simulink model "dynamic_range_compression"  (R2020b)
settings: Solver=FixedStepAuto  StartTime=0.0  StopTime=stop_time  RelTol=1e-3
values from neighbouring files (symbols this model uses):
  delay_memory_size = 2^system_delay_memory    [dynamic_range_compression_sim_init.m]    (also in test_FFT_to_gain_init.m)
  system_delay = gain_delay + accum_delay    [dynamic_range_compression_sim_init.m]    (also in test_FFT_to_gain_init.m)
libraries: hdlsllib x6
settings Model: Creator=t96f346  LastModifiedBy=conno
settings DataIOCC: SaveOutput=off  SaveTime=off  ReturnWorkspaceOutputs=off
settings ModelReferenceCC: ModelReferenceNumInstancesAllowed=Single

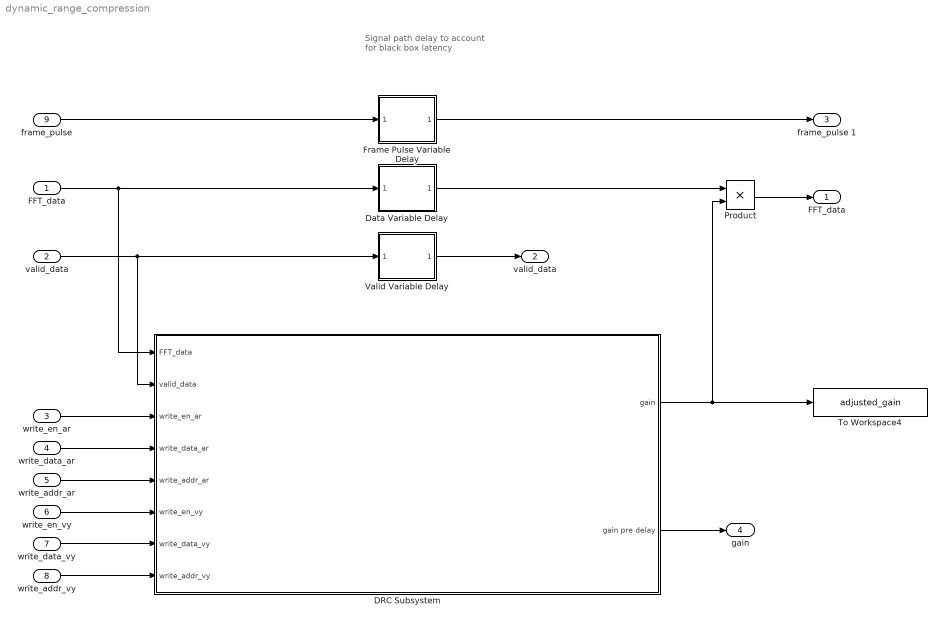
== system dynamic_range_compression ==
  note: Signal path delay to account for black box latency
  FFT_data : Inport  OutDataTypeStr=fixdt(1,40,32)  PortDimensions=[1 1]
      settings: SignalType=complex
  valid_data : Inport  Port=2  OutDataTypeStr=boolean  PortDimensions=[1 1]
  write_en_ar : Inport  Port=3  OutDataTypeStr=boolean  PortDimensions=[1 1]
  write_data_ar : Inport  Port=4  PortDimensions=[1 1]
  write_addr_ar : Inport  Port=5  OutDataTypeStr=uint8  PortDimensions=[1 1]
  write_en_vy : Inport  Port=6  OutDataTypeStr=boolean  PortDimensions=[1 1]
  write_data_vy : Inport  Port=7  OutDataTypeStr=fixdt(1,16,8)  PortDimensions=[1 1]
  write_addr_vy : Inport  Port=8  OutDataTypeStr=uint8  PortDimensions=[1 1]
  frame_pulse : Inport  Port=9  OutDataTypeStr=boolean  PortDimensions=[1 1]
  DRC Subsystem : Subsystem
  Data Variable Delay : Subsystem
  Frame Pulse Variable Delay : Subsystem
  Product : Product  OutDataTypeStr=fixdt(1,Wbits,Fbits)
  To Workspace4 : ToWorkspace  VariableName=adjusted_gain  SampleTime=-1
      settings: Save2DSignal=2-D array (concatenate along first dimension)
  Valid Variable Delay : Subsystem
  "FFT_data " : Outport  OutDataTypeStr=fixdt(1,40,32)  PortDimensions=1
      settings: SignalType=complex
  "valid_data " : Outport  Port=2  OutDataTypeStr=boolean  PortDimensions=1
  frame_pulse 1 : Outport  Port=3  OutDataTypeStr=boolean  PortDimensions=1
  gain : Outport  Port=4  PortDimensions=1
  wires:
  valid_data/1 -> Valid Variable Delay/1(data_in), DRC Subsystem/2(valid_data)
  FFT_data/1 -> Data Variable Delay/1(data_in), DRC Subsystem/1(FFT_data)
  Valid Variable Delay/1(rd_dout) -> "valid_data "/1
  write_en_ar/1 -> DRC Subsystem/3(write_en_ar)
  write_data_ar/1 -> DRC Subsystem/4(write_data_ar)
  write_addr_ar/1 -> DRC Subsystem/5(write_addr_ar)
  write_en_vy/1 -> DRC Subsystem/6(write_en_vy)
  write_data_vy/1 -> DRC Subsystem/7(write_data_vy)
  write_addr_vy/1 -> DRC Subsystem/8(write_addr_vy)
  DRC Subsystem/1("gain ") -> To Workspace4/1, Product/2
  Data Variable Delay/1(rd_dout) -> Product/1
  Product/1 -> "FFT_data "/1
  Frame Pulse Variable Delay/1(rd_dout) -> frame_pulse 1/1
  frame_pulse/1 -> Frame Pulse Variable Delay/1(data_in)
  DRC Subsystem/2(gain pre delay) -> gain/1

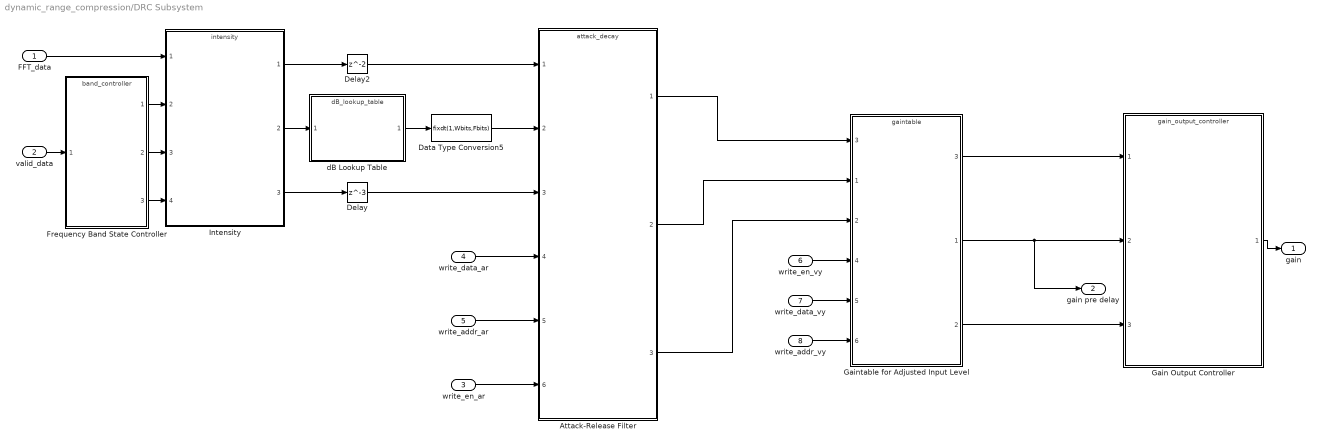
== system dynamic_range_compression/DRC Subsystem ==
  FFT_data : Inport
  valid_data : Inport  Port=2
  write_en_ar : Inport  Port=3
  write_data_ar : Inport  Port=4
  write_addr_ar : Inport  Port=5
  write_en_vy : Inport  Port=6
  write_data_vy : Inport  Port=7
  write_addr_vy : Inport  Port=8
  Attack-Release Filter : ModelReference  ModelNameDialog=attack_decay  SimulationMode=Normal  ModelReferenceVersion=2.75
  Data Type Conversion5 : DataTypeConversion  OutDataTypeStr=fixdt(1,Wbits,Fbits)
  Delay : Delay  DelayLength=3  InitialCondition=1
  Delay2 : Delay  InitialCondition=0
  Frequency Band State Controller : ModelReference  ModelNameDialog=band_controller.slx  SimulationMode=Normal  ModelReferenceVersion=2.34
  Gain Output Controller : ModelReference  ModelNameDialog=gain_output_controller.slx  SimulationMode=Normal  ModelReferenceVersion=2.28
  Gaintable for Adjusted Input Level : ModelReference  ModelNameDialog=gaintable  SimulationMode=Normal  ModelReferenceVersion=2.53
      settings: PortSchema="{\"entries\":[{\"content\":{\"sides\":[{\"content\":{\"connectorIds\":[\"In3\",\"In1\",\"In2\",\"In4\",\"In5\",\"In6\"]},\"type\":\"ConnectorPlacement.EquallySpacedRectSide\",\"uuid\":\"15a14a82-9bd7-4164-b619-b9bea276d1a9\"},{\"content\":{\"connectorIds\":[\"Out3\",\"Out1\",\"Out2\"],\"side\":\"RIGHT\"},\"type\":\"ConnectorPlacement.EquallySpacedRectSide\",\"uuid\":\"b762d0e2-66c7-466f-9495-f7c5ef747c3e\"},{\"content\":{\"connectorIds\":[],\"side\":\"TOP\"},\"type\":\"ConnectorPlacement.EquallySpacedRectSide\",\"uuid\":\"56b3a3d4-71ab-44aa-9541-48bc28b345d5\"},{\"content\":{\"connectorIds\":[],\"side\":\"HIDDEN\"},\"type\":\"ConnectorPlacement.EquallySpacedRectSide\",\"uuid\":\"17251429-5e91-446f-9fb8-583eb817a6ae\"}]},\"type\":\"ConnectorPlacement.EquallySpacedConnector\",\"uuid\":\"09e275fb-6840-46b7-a1cf-a56a9cd0acfa\"}],\"packageUris\":[\"http://schema.mathworks.com/mf0/Connector/R2020b\"],\"version\":\"1.0\"}"
  Intensity : ModelReference  ModelNameDialog=intensity  SimulationMode=Normal  ModelReferenceVersion=2.36
  dB Lookup Table : ModelReference  ModelNameDialog=dB_lookup_table  SimulationMode=Normal  ModelReferenceVersion=2.31
  "gain " : Outport
  gain pre delay : Outport  Port=2
  wires:
  Frequency Band State Controller/3 -> Intensity/4
  Gain Output Controller/1 -> "gain "/1
  valid_data/1 -> Frequency Band State Controller/1
  Intensity/2 -> dB Lookup Table/1
  FFT_data/1 -> Intensity/1
  Data Type Conversion5/1 -> Attack-Release Filter/2
  Gaintable for Adjusted Input Level/2 -> Gain Output Controller/3
  Frequency Band State Controller/1 -> Intensity/2
  Attack-Release Filter/2 -> Gaintable for Adjusted Input Level/1
  Delay/1 -> Attack-Release Filter/3
  Intensity/3 -> Delay/1
  Frequency Band State Controller/2 -> Intensity/3
  Delay2/1 -> Attack-Release Filter/1
  Intensity/1 -> Delay2/1
  Gaintable for Adjusted Input Level/1 -> Gain Output Controller/2, gain pre delay/1
  dB Lookup Table/1 -> Data Type Conversion5/1
  write_en_ar/1 -> Attack-Release Filter/6
  write_data_ar/1 -> Attack-Release Filter/4
  write_addr_ar/1 -> Attack-Release Filter/5
  Attack-Release Filter/3 -> Gaintable for Adjusted Input Level/2
  Attack-Release Filter/1 -> Gaintable for Adjusted Input Level/3
  Gaintable for Adjusted Input Level/3 -> Gain Output Controller/1
  write_en_vy/1 -> Gaintable for Adjusted Input Level/4
  write_data_vy/1 -> Gaintable for Adjusted Input Level/5
  write_addr_vy/1 -> Gaintable for Adjusted Input Level/6

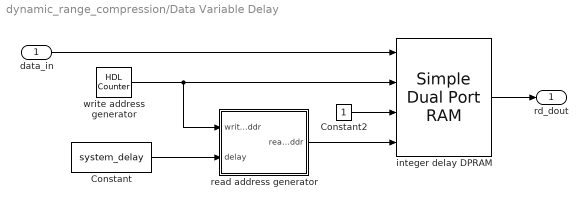
== system dynamic_range_compression/Data Variable Delay ==
  data_in : Inport
  Constant : Constant  Value=system_delay  OutDataTypeStr=uint8  SampleTime=-1
  Constant2 : Constant  OutDataTypeStr=Inherit: Inherit via back propagation  SampleTime=-1
  integer delay DPRAM : hdlsllib/HDL RAMs/Simple Dual Port RAM  ram_size=system_delay_memory
      settings: SourceProductBaseCode=SL
  read address generator : Subsystem
  write address generator : hdlsllib/Sources/HDL Counter  CountType=Count limited  CountInit=0  CountStep=1  CountMax=delay_memory_size - 1  CountFromType=Initial value  CountFrom=0  CountResetPort=off  CountLoadPort=off  CountEnbPort=off  CountDirPort=off  CountDataType=Unsigned  CountWordLen=system_delay_memory  CountFracLen=0  CountSampTime=-1
  rd_dout : Outport
  wires:
  read address generator/1(read_addr) -> integer delay DPRAM/4
  data_in/1 -> integer delay DPRAM/1
  Constant/1 -> read address generator/2(delay)
  integer delay DPRAM/1 -> rd_dout/1
  write address generator/1 -> read address generator/1(write_addr), integer delay DPRAM/2
  Constant2/1 -> integer delay DPRAM/3

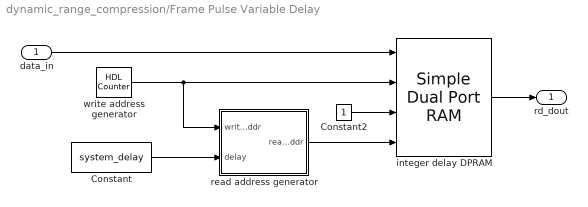
== system dynamic_range_compression/Frame Pulse Variable Delay ==
  data_in : Inport
  Constant : Constant  Value=system_delay  OutDataTypeStr=uint8  SampleTime=-1
  Constant2 : Constant  OutDataTypeStr=Inherit: Inherit via back propagation  SampleTime=-1
  integer delay DPRAM : hdlsllib/HDL RAMs/Simple Dual Port RAM  ram_size=system_delay_memory
      settings: SourceProductBaseCode=SL
  read address generator : Subsystem
  write address generator : hdlsllib/Sources/HDL Counter  CountType=Count limited  CountInit=0  CountStep=1  CountMax=delay_memory_size - 1  CountFromType=Initial value  CountFrom=0  CountResetPort=off  CountLoadPort=off  CountEnbPort=off  CountDirPort=off  CountDataType=Unsigned  CountWordLen=system_delay_memory  CountFracLen=0  CountSampTime=-1
  rd_dout : Outport
  wires:
  read address generator/1(read_addr) -> integer delay DPRAM/4
  data_in/1 -> integer delay DPRAM/1
  Constant/1 -> read address generator/2(delay)
  integer delay DPRAM/1 -> rd_dout/1
  write address generator/1 -> read address generator/1(write_addr), integer delay DPRAM/2
  Constant2/1 -> integer delay DPRAM/3

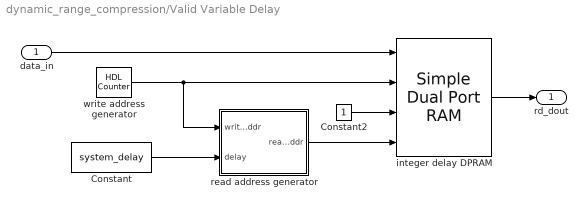
== system dynamic_range_compression/Valid Variable Delay ==
  data_in : Inport
  Constant : Constant  Value=system_delay  OutDataTypeStr=uint8  SampleTime=-1
  Constant2 : Constant  OutDataTypeStr=Inherit: Inherit via back propagation  SampleTime=-1
  integer delay DPRAM : hdlsllib/HDL RAMs/Simple Dual Port RAM  ram_size=system_delay_memory
      settings: SourceProductBaseCode=SL
  read address generator : Subsystem
  write address generator : hdlsllib/Sources/HDL Counter  CountType=Count limited  CountInit=0  CountStep=1  CountMax=delay_memory_size - 1  CountFromType=Initial value  CountFrom=0  CountResetPort=off  CountLoadPort=off  CountEnbPort=off  CountDirPort=off  CountDataType=Unsigned  CountWordLen=system_delay_memory  CountFracLen=0  CountSampTime=-1
  rd_dout : Outport
  wires:
  read address generator/1(read_addr) -> integer delay DPRAM/4
  data_in/1 -> integer delay DPRAM/1
  Constant/1 -> read address generator/2(delay)
  integer delay DPRAM/1 -> rd_dout/1
  write address generator/1 -> read address generator/1(write_addr), integer delay DPRAM/2
  Constant2/1 -> integer delay DPRAM/3

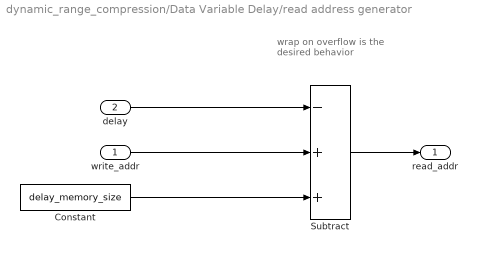
== system dynamic_range_compression/Data Variable Delay/read address generator ==
  note: wrap on overflow is the desired behavior
  write_addr : Inport
  delay : Inport  Port=2
  Constant : Constant  Value=delay_memory_size  SampleTime=-1
  Subtract : Sum  Inputs=-++  OutDataTypeStr=Inherit: Inherit via back propagation
  read_addr : Outport  VectorParamsAs1DForOutWhenUnconnected=off
  wires:
  Constant/1 -> Subtract/3
  delay/1 -> Subtract/1
  write_addr/1 -> Subtract/2
  Subtract/1 -> read_addr/1

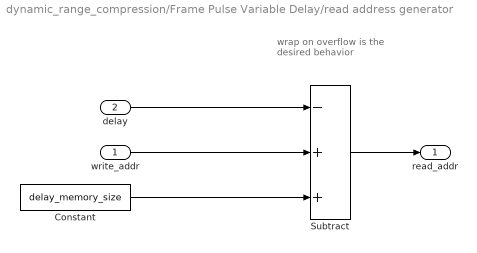
== system dynamic_range_compression/Frame Pulse Variable Delay/read address generator ==
  note: wrap on overflow is the desired behavior
  write_addr : Inport
  delay : Inport  Port=2
  Constant : Constant  Value=delay_memory_size  SampleTime=-1
  Subtract : Sum  Inputs=-++  OutDataTypeStr=Inherit: Inherit via back propagation
  read_addr : Outport  VectorParamsAs1DForOutWhenUnconnected=off
  wires:
  Constant/1 -> Subtract/3
  delay/1 -> Subtract/1
  write_addr/1 -> Subtract/2
  Subtract/1 -> read_addr/1

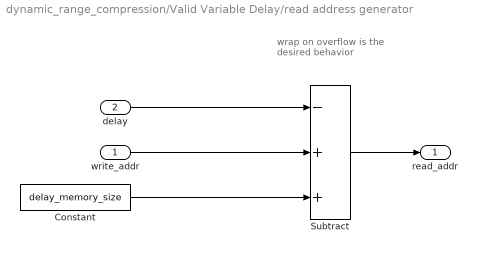
== system dynamic_range_compression/Valid Variable Delay/read address generator ==
  note: wrap on overflow is the desired behavior
  write_addr : Inport
  delay : Inport  Port=2
  Constant : Constant  Value=delay_memory_size  SampleTime=-1
  Subtract : Sum  Inputs=-++  OutDataTypeStr=Inherit: Inherit via back propagation
  read_addr : Outport  VectorParamsAs1DForOutWhenUnconnected=off
  wires:
  Constant/1 -> Subtract/3
  delay/1 -> Subtract/1
  write_addr/1 -> Subtract/2
  Subtract/1 -> read_addr/1
